simulink model "Diagrama_edificio_CIESOL"  (R2019b)
settings: Solver=VariableStepAuto  StartTime=0.0  StopTime=10.0  RelTol=1e-3
libraries: Libreria x11
settings Model: Creator=PC-01  LastModifiedBy=PC-01

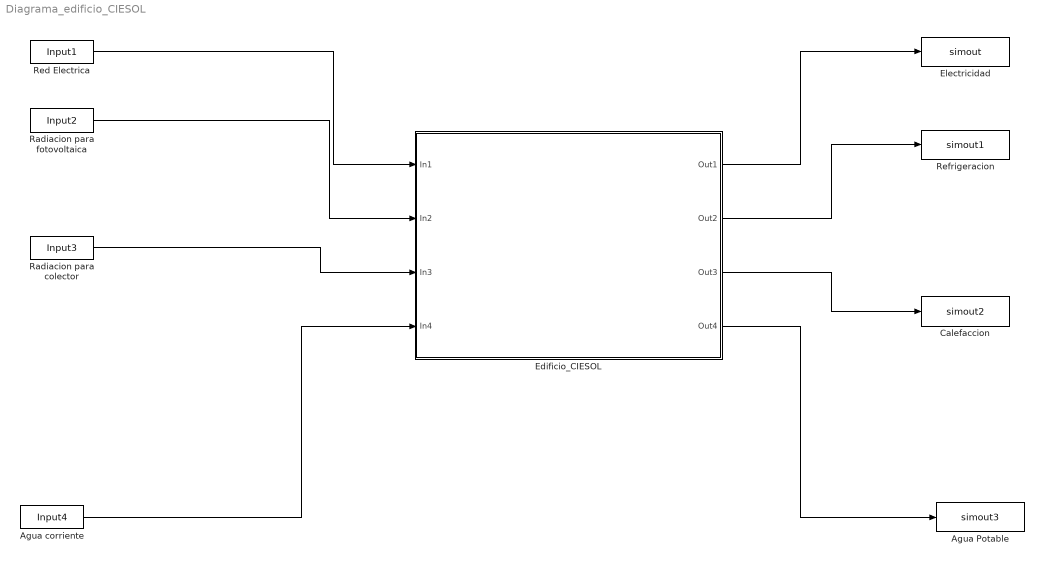
== system Diagrama_edificio_CIESOL ==
  Agua Potable : ToWorkspace  VariableName=simout3  SaveFormat=Timeseries  SampleTime=-1
  Agua corriente : FromWorkspace  VariableName=Input4  SampleTime=0
  Calefaccion : ToWorkspace  VariableName=simout2  SaveFormat=Timeseries  SampleTime=-1
  Edificio_CIESOL : Subsystem
  Electricidad : ToWorkspace  VariableName=simout  SaveFormat=Timeseries  SampleTime=-1
  Radiacion para colector : FromWorkspace  VariableName=Input3  SampleTime=0
  Radiacion para fotovoltaica : FromWorkspace  VariableName=Input2  SampleTime=0
  Red Electrica : FromWorkspace  VariableName=Input1  SampleTime=0
  Refrigeracion : ToWorkspace  VariableName=simout1  SaveFormat=Timeseries  SampleTime=-1
  wires:
  Red Electrica/1 -> Edificio_CIESOL/1(In1)
  Radiacion para fotovoltaica/1 -> Edificio_CIESOL/2(In2)
  Radiacion para colector/1 -> Edificio_CIESOL/3(In3)
  Agua corriente/1 -> Edificio_CIESOL/4(In4)
  Edificio_CIESOL/1(Out1) -> Electricidad/1
  Edificio_CIESOL/2(Out2) -> Refrigeracion/1
  Edificio_CIESOL/3(Out3) -> Calefaccion/1
  Edificio_CIESOL/4(Out4) -> Agua Potable/1

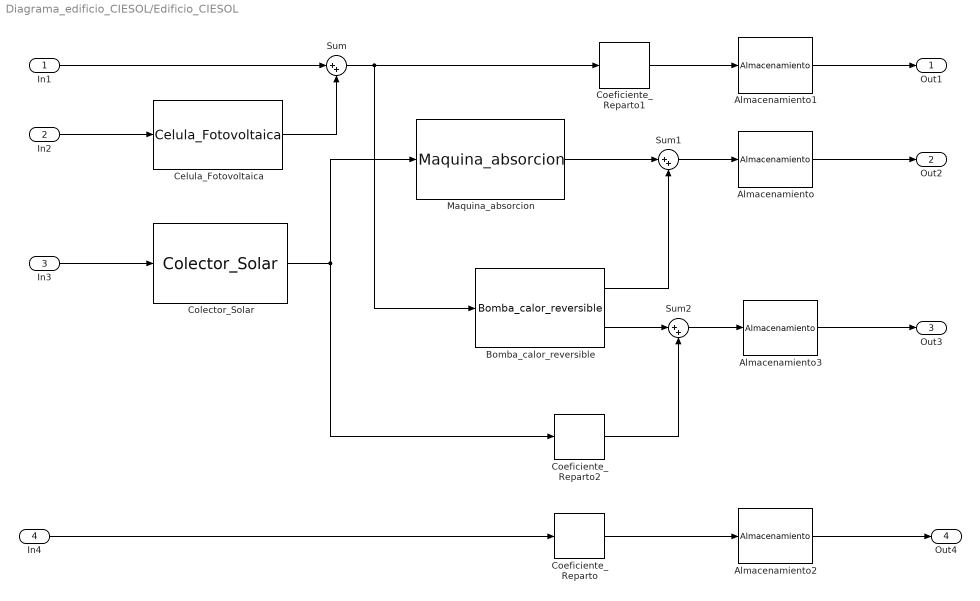
== system Diagrama_edificio_CIESOL/Edificio_CIESOL ==
  In1 : Inport
  In2 : Inport  Port=2
  In3 : Inport  Port=3
  In4 : Inport  Port=4
  Almacenamiento : Libreria/Almacenamiento  Up2=20.9  Low2=0  r_c=0.9  Up=20.9  Low=0  r_d=0.9  Up1=29  Low1=0  almacenamiento_inicial=0  cpa=0.02  almacenamiento_on=on
  Almacenamiento1 : Libreria/Almacenamiento  Up2=1000  Low2=0  r_c=1  Up=1000  Low=0  r_d=1  Up1=1000  Low1=0  almacenamiento_inicial=0  cpa=1  almacenamiento_on=on
  Almacenamiento2 : Libreria/Almacenamiento  Up2=1000  Low2=0  r_c=1  Up=1000  Low=0  r_d=1  Up1=1000  Low1=0  almacenamiento_inicial=0  cpa=1  almacenamiento_on=on
  Almacenamiento3 : Libreria/Almacenamiento  Up2=125.4  Low2=0  r_c=0.9  Up=125.4  Low=0  r_d=0.9  Up1=174.2  Low1=0  almacenamiento_inicial=0  cpa=0.06  almacenamiento_on=on
  Bomba_calor_reversible : Libreria/Bomba_calor_reversible  efficiency=[2.9 3.1]  dispatch_factor=1  T_muestreo=T_muestreo  Max_in=26.5  Min_in=0  Max_out=[76.4 82.6]  Salida_Binaria=[1 0]
  Celula_Fotovoltaica : Libreria/Celula_Fotovoltaica  efficiency=0.1207  dispatch_factor=1  T_muestreo=T_muestreo  Max_in=68.376  Max_out=8.2584343
  Coeficiente_Reparto : Libreria/Coeficiente_Reparto  dispatch_factor=1  Tm=T_muestreo  Max_out=inf  Max_in=inf  efficiency=1
  Coeficiente_Reparto1 : Libreria/Coeficiente_Reparto  dispatch_factor=alfa1  Tm=T_muestreo  Max_out=inf  Max_in=inf  efficiency=1
  Coeficiente_Reparto2 : Libreria/Coeficiente_Reparto  dispatch_factor=alfa2  Tm=T_muestreo  Max_out=inf  Max_in=inf  efficiency=1
  Colector_Solar : Libreria/Colector_Solar  efficiency=[0.211]  dispatch_factor=1  T_muestreo=T_muestreo  Max_in=1200  Max_out=2000
  Maquina_absorcion : Libreria/Maquina_absorcion  efficiency=0.7  dispatch_factor=alfa2  Tm=T_muestreo  Min_in=0  Max_in=100  Max_out=70
  Sum : Sum  Inputs=|++
  Sum1 : Sum  Inputs=|++
  Sum2 : Sum  Inputs=|++
  Out1 : Outport
  Out2 : Outport  Port=2
  Out3 : Outport  Port=3
  Out4 : Outport  Port=4
  wires:
  Bomba_calor_reversible/1 -> Sum1/2
  Bomba_calor_reversible/2 -> Sum2/1
  Almacenamiento1/1 -> Out1/1
  Maquina_absorcion/1 -> Sum1/1
  Coeficiente_Reparto2/1 -> Sum2/2
  Celula_Fotovoltaica/1 -> Sum/2
  Coeficiente_Reparto1/1 -> Almacenamiento1/1
  Almacenamiento3/1 -> Out3/1
  Colector_Solar/1 -> Coeficiente_Reparto2/1, Maquina_absorcion/1
  Sum1/1 -> Almacenamiento/1
  Sum/1 -> Bomba_calor_reversible/1, Coeficiente_Reparto1/1
  In2/1 -> Celula_Fotovoltaica/1
  Sum2/1 -> Almacenamiento3/1
  Coeficiente_Reparto/1 -> Almacenamiento2/1
  In3/1 -> Colector_Solar/1
  Almacenamiento/1 -> Out2/1
  In1/1 -> Sum/1
  In4/1 -> Coeficiente_Reparto/1
  Almacenamiento2/1 -> Out4/1
